simulink model "Lab4Simulink"  (R2018a)
settings: Solver=VariableStepAuto  StartTime=0.0  StopTime=10  RelTol=1e-6
libraries: simulink x1
settings Model: Creator=rahul  LastModifiedBy=rahul

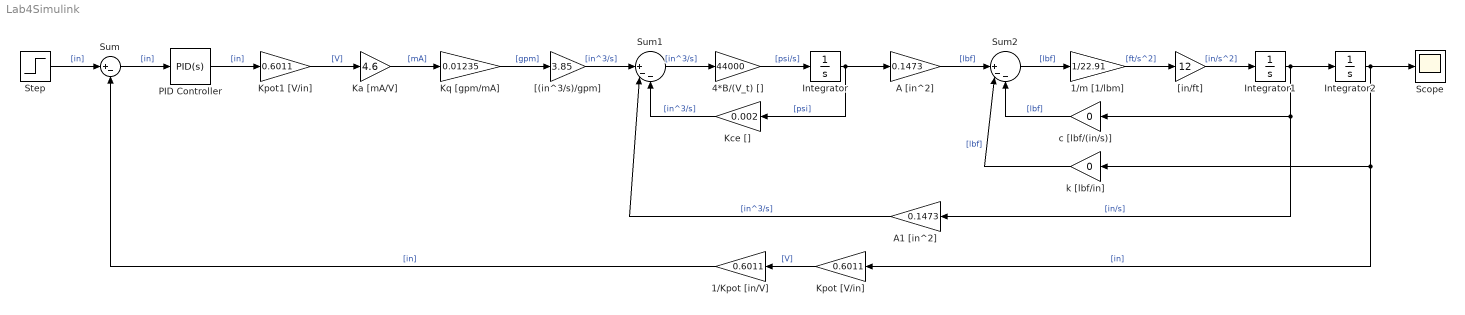
== system Lab4Simulink ==
  1/Kpot [in/V] : Gain  Gain=0.6011
  1/m [1/lbm] : Gain  Gain=1/22.91
  4*B/(V_t) [] : Gain  Gain=44000
  A [in^2] : Gain  Gain=0.1473
  A1 [in^2] : Gain  Gain=0.1473
  Integrator : Integrator
  Integrator1 : Integrator
  Integrator2 : Integrator
  Ka [mA/V] : Gain  Gain=4.6
  Kce [] : Gain  Gain=0.002
  Kpot [V/in] : Gain  Gain=0.6011
  Kpot1 [V/in] : Gain  Gain=0.6011
  Kq [gpm/mA] : Gain  Gain=0.01235
  "PID Controller " : simulink/Continuous/PID Controller  Controller=PID  TimeDomain=Continuous-time  SampleTime=-1  IntegratorMethod=Forward Euler  FilterMethod=Forward Euler  Form=Parallel  UseFilter=on  ControllerParametersSource=internal  P=300  I=0  D=0  N=100  InitialConditionSource=internal  InitialConditionForIntegrator=0  InitialConditionForFilter=0  ExternalReset=none  LimitOutput=off  UpperSaturationLimit=inf  LowerSaturationLimit=-inf  LinearizeAsGain=on  AntiWindupMode=none  Kb=1  TrackingMode=off  Kt=1  PParamMin=[]  PParamMax=[]  IParamMin=[]  IParamMax=[]  DParamMin=[]  DParamMax=[]  NParamMin=[]  NParamMax=[]  KbParamMin=[]  KbParamMax=[]  KtParamMin=[]  KtParamMax=[]  POutMin=[]  POutMax=[]  IOutMin=[]  IOutMax=[]  DOutMin=[]  DOutMax=[]  NOutMin=[]  NOutMax=[]  KbOutMin=[]  KbOutMax=[]  KtOutMin=[]  KtOutMax=[]  IntegratorOutMin=[]  IntegratorOutMax=[]  FilterOutMin=[]  FilterOutMax=[]  SumOutMin=[]  SumOutMax=[]  SumI1OutMin=[]  SumI1OutMax=[]  SumI2OutMin=[]  SumI2OutMax=[]  SumI3OutMin=[]  SumI3OutMax=[]  SumDOutMin=[]  SumDOutMax=[]  SaturationOutMin=[]  SaturationOutMax=[]  IntegratorContinuousStateAttributes=''  IntegratorStateMustResolveToSignalObject=off  IntegratorRTWStateStorageClass=Auto  FilterContinuousStateAttributes=''  FilterStateMustResolveToSignalObject=off  FilterRTWStateStorageClass=Auto  DifferentiatorICPrevScaledInput=0  DifferentiatorOutMin=[]  DifferentiatorOutMax=[]  FilterDiffOutCoefMin=[]  FilterDiffOutCoefMax=[]  SumDenOutMin=[]  SumDenOutMax=[]  SumNumOutMin=[]  SumNumOutMax=[]  ReciprocalOutMin=[]  ReciprocalOutMax=[]  DivideOutMin=[]  DivideOutMax=[]  TunerSelectOption=Transfer Function Based (PID Tuner App)
  Scope : Scope
  Step : Step  SampleTime=0
  Sum : Sum  Inputs=|+-
  Sum1 : Sum  Inputs=||+--
  Sum2 : Sum  Inputs=||+--
  "[(in^3/s)/gpm]" : Gain  Gain=3.85
  "[in/ft]" : Gain  Gain=12
  c [lbf/(in/s)] : Gain  Gain=0
  k [lbf/in] : Gain  Gain=0
  wires:
  Step/1 -> Sum/1  "[in]"
  Kpot1 [V/in]/1 -> Ka [mA/V]/1  "[V]"
  Ka [mA/V]/1 -> Kq [gpm/mA]/1  "[mA]"
  Sum1/1 -> 4*B/(V_t) []/1  "[in^3/s]"
  4*B/(V_t) []/1 -> Integrator/1  "[psi/s]"
  Integrator/1 -> Kce []/1, A [in^2]/1  "[psi]"
  A [in^2]/1 -> Sum2/1  "[lbf]"
  Sum2/1 -> 1/m [1/lbm]/1  "[lbf]"
  Integrator1/1 -> A1 [in^2]/1, c [lbf/(in/s)]/1, Integrator2/1  "[in/s]"
  Integrator2/1 -> Kpot [V/in]/1, k [lbf/in]/1, Scope/1  "[in]"
  c [lbf/(in/s)]/1 -> Sum2/3  "[lbf]"
  k [lbf/in]/1 -> Sum2/2  "[lbf]"
  A1 [in^2]/1 -> Sum1/2  "[in^3/s]"
  Kce []/1 -> Sum1/3  "[in^3/s]"
  Kpot [V/in]/1 -> 1/Kpot [in/V]/1  "[V]"
  1/Kpot [in/V]/1 -> Sum/2  "[in]"
  "PID Controller "/1 -> Kpot1 [V/in]/1  "[in]"
  Sum/1 -> "PID Controller "/1  "[in]"
  "[(in^3/s)/gpm]"/1 -> Sum1/1  "[in^3/s]"
  Kq [gpm/mA]/1 -> "[(in^3/s)/gpm]"/1  "[gpm]"
  1/m [1/lbm]/1 -> "[in/ft]"/1  "[ft/s^2]"
  "[in/ft]"/1 -> Integrator1/1  "[in/s^2]"
